simulink model "dekf_estimate_attempt_3_early"  (R2021a)
settings: Solver=VariableStepAuto  StartTime=0.0  StopTime=time_est_1  RelTol=1e-3
values from neighbouring files (symbols this model uses):
  Delta = block.DialogPrm(1).Data    [battery_dual_ekf.m]    (also in battery_dual_ekf_2.m; battery_dual_ekf_early.m; init_dekf_3.m = 0.008; kalman_validate.m)
settings Model: Creator=saleh  LastModifiedBy=saleh

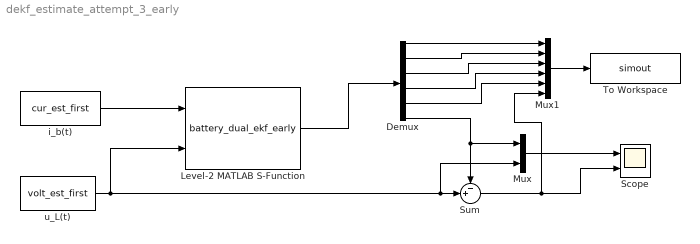
== system dekf_estimate_attempt_3_early ==
  Demux : Demux  Outputs=6
  Level-2 MATLAB S-Function : M-S-Function  FunctionName=battery_dual_ekf_early  Parameters=Delta, x0, P0, a, Z_b_k, W_k, Qe
  Mux : Mux  Inputs=2
  Mux1 : Mux  Inputs=6
  Scope : Scope  NumInputPorts=2
  Sum : Sum  Inputs=-+|
  To Workspace : ToWorkspace  VariableName=simout  SampleTime=-1
  i_b(t) : FromWorkspace  VariableName=cur_est_first  SampleTime=Delta
  u_L(t) : FromWorkspace  VariableName=volt_est_first  SampleTime=Delta
  wires:
  i_b(t)/1 -> Level-2 MATLAB S-Function/1
  u_L(t)/1 -> Level-2 MATLAB S-Function/2, Mux/2, Sum/2
  Level-2 MATLAB S-Function/1 -> Demux/1
  Demux/6 -> Mux/1, Sum/1
  Sum/1 -> Mux1/6, Scope/2
  Mux/1 -> Scope/1
  Demux/1 -> Mux1/1
  Demux/2 -> Mux1/2
  Demux/3 -> Mux1/3
  Demux/4 -> Mux1/4
  Demux/5 -> Mux1/5
  Mux1/1 -> To Workspace/1
